simulink model "hysteresis_ctrl2222"  (R2021a)
settings: Solver=VariableStepAuto  StartTime=0.0  StopTime=0.1  RelTol=1e-3
libraries: spsCurrentMeasurementLib x1, spsDiodeLib x1, spsIGBTDiodeLib x1, spsSeriesRLCBranchLib x1, spsVoltageMeasurementLib x1, spsDCVoltageSourceLib x1, spspowerguiLib x1
settings Model: Creator=Himel Khan  LastModifiedBy=User

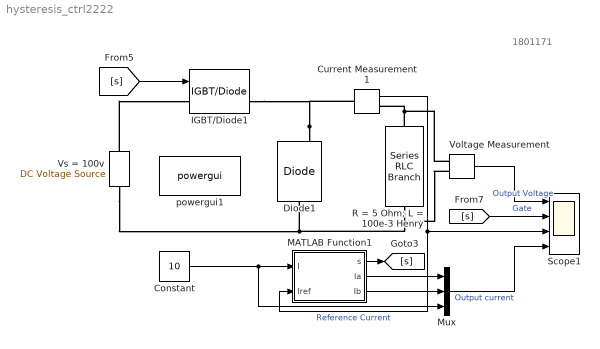
== system hysteresis_ctrl2222 ==
  note: 1801171
  Constant : Constant  Value=10
  Current Measurement1 : spsCurrentMeasurementLib/Current Measurement  PhasorSimulation=off  OutputType=Complex  PSBequivalent=0
  Diode1 : spsDiodeLib/Diode  Ron=0.001  Lon=0  Vf=0.8  IC=0  UseSnubber=0  Rs=500  Cs=250e-9  Measurements=on
  IGBT/Diode1 : spsIGBTDiodeLib/IGBT//Diode  Ron=1e-3  Rs=1e5  Cs=inf  Measurements=on
  MATLAB Function1 : MATLAB Function  TreatAsAtomicUnit=on
  Mux : Mux  Inputs=3
  R = 5 Ohm; L = 100e-3 Henry : spsSeriesRLCBranchLib/Series RLC Branch  LConnTagsString=__new0  RConnTagsString=__new0  BranchType=RL  Resistance=5  Inductance=100e-3  SetiL0=off  InitialCurrent=0  Capacitance=1e-6  Setx0=off  InitialVoltage=0  Measurements=None
  Scope1 : Scope  NumInputPorts=4
  Voltage Measurement : spsVoltageMeasurementLib/Voltage Measurement  PhasorSimulation=off  OutputType=Complex  PSBequivalent=0
  Vs = 100v : spsDCVoltageSourceLib/DC Voltage Source  Amplitude=100  Measurements=None
  powergui1 : spspowerguiLib/powergui  Priority=1  SimulationMode=Discrete  SampleTime=50e-6  frequency=60  Iterations=50  frequencyindice=0  Pbase=100e6  ErrMax=1e-4  UnitsV=kV  UnitsW=MW  buscounter=0  FunctionMessages=off  echomessages=off  EnableUseOfTLC=off  CurrentSourceSwitches=off  DisableSnubberDevices=off  DisableRonSwitches=off  DisableVfSwitches=off  DisplayEquations=off  AutomaticDiscreteSolvers=off  SolverType=Tustin/Backward Euler (TBE)  Interpol=off  ExternalGateDelay=off  methode=off  Ts=100  x0status=blocks  SPID=on  SwTol=0  HookPort=off  NonlinearTolerance=1e-4  nMaxIteration=100  ContinueOnMaxIteration=off  RestoreLinks=warning  ResistiveCurrentMeasurement=off  Frange=[0:2:500]  Ylog=off  Xlog=on  ShowGrid=off  save=off  variable=ZData  structure=0  ZoomFFT=off  StartTime=0.0  cycles=1  DisplayStyle=1  fundamental=60  FreqAxis=off  MaxFrequency=1000  frequencyindicesteady=1  RmsSteady=1  display=off
  wires:
  MATLAB Function1/1(s) -> [s]
  [s] -> IGBT/Diode1/1
  [s] -> Scope1/2  "Gate"
  Current Measurement1/1 -> MATLAB Function1/2(Iref), Scope1/3  "Reference Current"
  Constant/1 -> Mux/3, MATLAB Function1/1(I)
  MATLAB Function1/2(Ia) -> Mux/1
  MATLAB Function1/3(Ib) -> Mux/2
  Mux/1 -> Scope1/4  "Output current"
  Voltage Measurement/1 -> Scope1/1  "Output Voltage"
  connections:
  Diode1/RConn1 -- IGBT/Diode1/RConn1 -- Current Measurement1/LConn1
  Vs = 100v/LConn1 -- Voltage Measurement/LConn2 -- R = 5 Ohm; L = 100e-3 Henry/RConn1 -- Diode1/LConn1
  R = 5 Ohm; L = 100e-3 Henry/LConn1 -- Voltage Measurement/LConn1 -- Current Measurement1/RConn1
  Vs = 100v/RConn1 -- IGBT/Diode1/LConn1

== matlab function hysteresis_ctrl2222/MATLAB Function1 ==
  data: I input; s output; Iref input; Ia output; Ib output
function [s,Ia,Ib]  = fcn(I,Iref)
persistent d
if isempty(d),d=1;end
e=1
Ia=I+e;
Ib=I-e;
if Iref>Ia
    d =0;
elseif Iref<Ib
    d=1;
else
    d=d;
end
s=d
end
